simulink model "BoostOpenLoopTest"  (R2020a)
settings: Solver=ode15s  StartTime=0.0  StopTime=0.05  RelTol=1e-3
undefined symbols (not defined in the file): Down, Fsw, GateVoltage, PWMResolution, Up
libraries: eeGeneralControl x2, ee_lib x2, fl_lib x1, nesl_utility x1
settings Model: Creator=ykamatan  LastModifiedBy=ykamatan
settings SolverCC: MaxConsecutiveMinStep=10

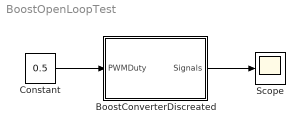
== system BoostOpenLoopTest ==
  BoostConverterDiscreated : Subsystem
  Constant : Constant  Value=0.5
  Scope : Scope
  wires:
  Constant/1 -> BoostConverterDiscreated/1(PWMDuty)
  BoostConverterDiscreated/1(Signals) -> Scope/1

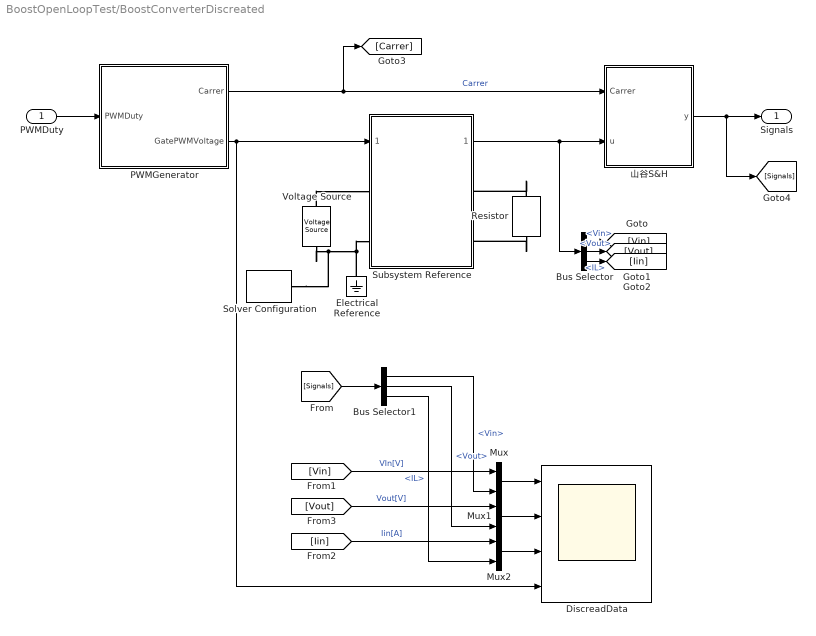
== system BoostOpenLoopTest/BoostConverterDiscreated ==
  PWMDuty : Inport
  Bus Selector : BusSelector  OutputSignals=Vin,Vout,IL
  Bus Selector1 : BusSelector  OutputSignals=Vin,Vout,IL
  DiscreadData : Scope  NumInputPorts=4
  Electrical Reference : fl_lib/Electrical/Electrical Elements/Electrical Reference
  Mux : Mux  Inputs=2
  Mux1 : Mux  Inputs=2
  Mux2 : Mux  Inputs=2
  PWMGenerator : Subsystem
  Resistor : ee_lib/Passive/Resistor  R=40 Ohm  R_tol=5  enable_R_tol=0  tol_distribution=1  nSigma=4  enable_operating_limits=0  operating_limit_action=2  max_working_voltage=100 V  power_rating=1 W  enable_faults=0  fault_action=1  R_faulted=inf Ohm  enable_temporal_fault=0  t_fault=1 s  enable_behavioral_fault=0  max_permissible_current=1 A  t_fail_on_current=1 s  noise_mode=0  sample_time=1e-3 s  repeatability=1  auto_seed=804803381  user_seed=0  Tdevice=25 degC  alpha=3.93e-3 1/K  Tmeas=25 degC  thermal_mass=100 J/K  power_derating_T1=70 degC  power_derating_T2=155 degC  operating_temperature_range_vec=[-50, 150] degC  temperature_specify=off  temperature_priority=High  temperature=298.15 K  temperature_nominal_specify=off  temperature_nominal_unit=K  temperature_nominal_value=1
  Solver Configuration : nesl_utility/Solver Configuration  PhysicalDomain=network_engine_domain  SubClassName=solver  LeftPortType=input  RightPortType=generic  Tones=[]  Harmonics=[]  SimulateNoise=off  Profile=off  UseLocalSampling=off  EnableSwitchedLinearOptims=on  FrequencyDomain=off  UseCCode=off  RelTol=0.001  AbsTol=1e-06  MinStep=1e-09  ToWorkspace=off  RevertToSquareIcSolve=off  NumHomotopyIterations=100  PhasorMode=off  PhasorModeNumHarmonics=1  DoDC=off  ResidualTolerance=1e-09  UseLocalSolver=off  LocalSolverChoice=NE_BACKWARD_EULER_ADVANCER  LocalSolverSampleTime=0.001  DoFixedCost=off  MaxNonlinIter=3  MaxModeIter=2  LinearAlgebra=auto  EquationFormulation=NE_TIME_EF  DelaysMemoryBudget=1024  AutomaticFiltering=on  FilteringTimeConstant=0.001  PartitionStorageMethod=AS_NEEDED  PartitionMemoryBudget=1024  PartitionMethod=ROBUST
  Subsystem Reference : Subsystem  ReferencedSubsystem=BoostConverter
  Voltage Source : ee_lib/Sources/Voltage Source  dc_voltage=100 V  ac_voltage=0 V  ac_shift=0 rad  ac_frequency=60 Hz  noise_mode=0  PSD=0 V^2/Hz  repeatability=1  auto_seed=1970210993  user_seed=0  sample_time=1e-3 s  i_specify=off  i_priority=None  i=0 A  i_nominal_specify=off  i_nominal_unit=A  i_nominal_value=1  v_specify=off  v_priority=None  v=0 V  v_nominal_specify=off  v_nominal_unit=V  v_nominal_value=1
  山谷S&H : Subsystem
  Signals : Outport
  wires:
  PWMGenerator/2(GatePWMVoltage) -> Subsystem Reference/1, DiscreadData/4
  [Vout] -> Mux1/1  "Vout[V]"
  [Vin] -> Mux/1  "VIn[V]"
  PWMDuty/1 -> PWMGenerator/1(PWMDuty)
  [Iin] -> Mux2/1  "Iin[A]"
  PWMGenerator/1(Carrer) -> 山谷S&H/1(Carrer), [Carrer]  "Carrer"
  Bus Selector/2 -> [Vout]  "<Vout>"
  Subsystem Reference/1 -> 山谷S&H/2(u), Bus Selector/1
  Bus Selector/1 -> [Vin]  "<Vin>"
  山谷S&H/1(y) -> Signals/1, [Signals]
  Bus Selector/3 -> [Iin]  "<IL>"
  Bus Selector1/1 -> Mux/2  "<Vin>"
  Bus Selector1/2 -> Mux1/2  "<Vout>"
  Bus Selector1/3 -> Mux2/2  "<IL>"
  Mux2/1 -> DiscreadData/3
  Mux1/1 -> DiscreadData/2
  Mux/1 -> DiscreadData/1
  [Signals] -> Bus Selector1/1
  connections:
  Voltage Source/RConn1 -- Solver Configuration/RConn1 -- Electrical Reference/LConn1 -- Subsystem Reference/LConn2
  Voltage Source/LConn1 -- Subsystem Reference/LConn1
  Resistor/RConn1 -- Subsystem Reference/RConn2
  Resistor/LConn1 -- Subsystem Reference/RConn1

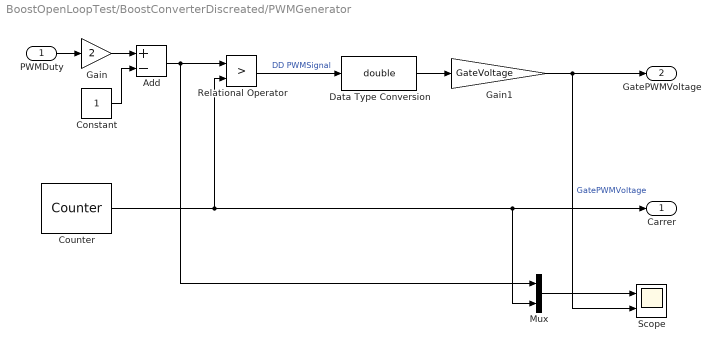
== system BoostOpenLoopTest/BoostConverterDiscreated/PWMGenerator ==
  PWMDuty : Inport
  Add : Sum  Inputs=+-
  Constant : Constant
  Counter : eeGeneralControl/Counter  CarrCount=Up-Down  Range=[-1 1]  Tper=1/Fsw/2  Tdelay=0  Ts=1/Fsw*PWMResolution
      settings: SourceProductBaseCode=PS
  Data Type Conversion : DataTypeConversion  OutDataTypeStr=double
  Gain : Gain  Gain=2
  Gain1 : Gain  Gain=GateVoltage
  Mux : Mux  Inputs=2
  Relational Operator : RelationalOperator  Operator=>  OutDataTypeStr=boolean  RndMeth=Simplest
  Scope : Scope  NumInputPorts=2
  Carrer : Outport
  GatePWMVoltage : Outport  Port=2
  wires:
  Add/1 -> Relational Operator/1, Mux/1
  Constant/1 -> Add/2
  Counter/1 -> Carrer/1, Mux/2, Relational Operator/2
  PWMDuty/1 -> Gain/1
  Gain/1 -> Add/1
  Relational Operator/1 -> Data Type Conversion/1  "DD PWMSignal"
  Data Type Conversion/1 -> Gain1/1
  Gain1/1 -> GatePWMVoltage/1, Scope/2  "GatePWMVoltage"
  Mux/1 -> Scope/1

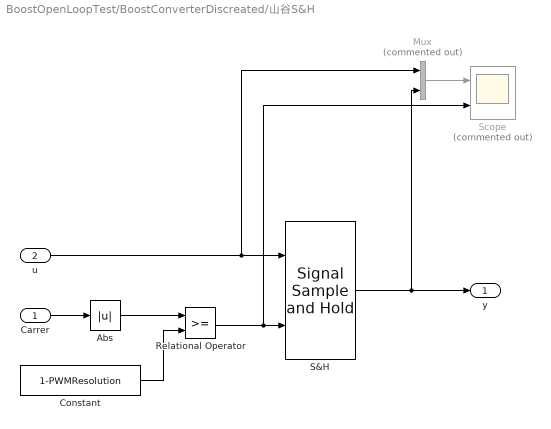
== system BoostOpenLoopTest/BoostConverterDiscreated/山谷S&H ==
  Carrer : Inport
  u : Inport  Port=2
  Abs : Abs
  Constant : Constant  Value=1-PWMResolution
  Mux : Mux  Commented=on  Inputs=2
  Relational Operator : RelationalOperator  OutDataTypeStr=boolean  ZeroCross=off  RndMeth=Simplest
  S&H : eeGeneralControl/Signal Sample and Hold  LabelModeActiveChoice=Discrete  x0=0  Ts=-1
      settings: SourceProductBaseCode=PS
  Scope : Scope  Commented=on  NumInputPorts=2
  y : Outport
  wires:
  Relational Operator/1 -> Scope/2, S&H/2
  S&H/1 -> Mux/2, y/1
  u/1 -> Mux/1, S&H/1
  Carrer/1 -> Abs/1
  Mux/1 -> Scope/1
  Abs/1 -> Relational Operator/1
  Constant/1 -> Relational Operator/2
